simulink model "model1"  (R2023a)
settings: Solver=VariableStepAuto  StartTime=0.0  StopTime=40  RelTol=1e-3
settings Model: Creator=evdokiiagalkina  LastModifiedBy=evdokiiagalkina

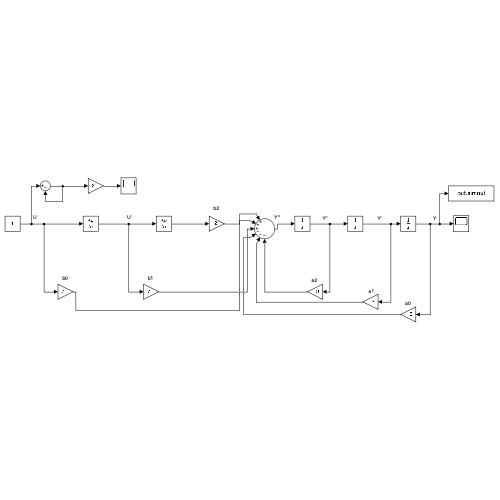
[thumbnail: Simulink's stored preview of the top-level diagram]
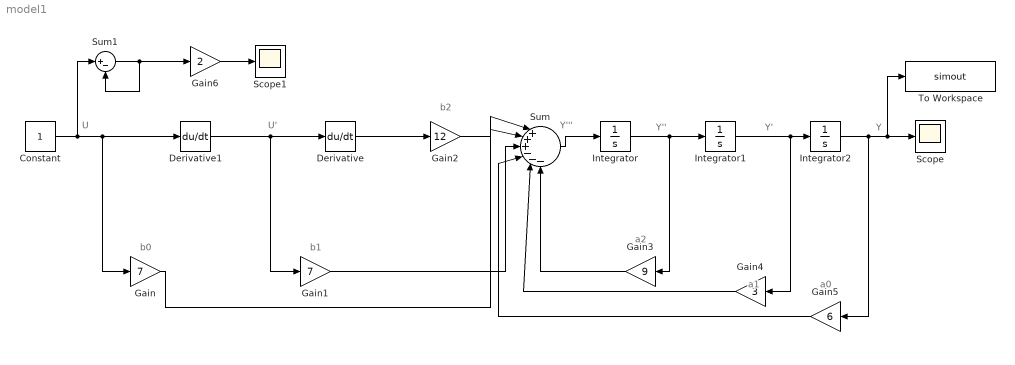
== system model1 ==
  note: Y''
  note: Y'''
  note: U'
  note: b0
  note: U
  note: b1
  note: b2
  note: Y'
  note: Y
  note: a2
  note: a1
  note: a0
  Constant : Constant
  Derivative : Derivative
  Derivative1 : Derivative
  Gain : Gain  Gain=7
  Gain1 : Gain  Gain=7
  Gain2 : Gain  Gain=12
  Gain3 : Gain  Gain=9
  Gain4 : Gain  Gain=3
  Gain5 : Gain  Gain=6
  Gain6 : Gain  Gain=2
  Integrator : Integrator
  Integrator1 : Integrator
  Integrator2 : Integrator
  Scope : Scope
  Scope1 : Scope
  Sum : Sum  Inputs=|+++---
  Sum1 : Sum  Inputs=|+-
  To Workspace : ToWorkspace  VariableName=simout  SaveFormat=Timeseries  SampleTime=-1
  wires:
  Sum/1 -> Integrator/1
  Derivative1/1 -> Derivative/1, Gain1/1
  Derivative/1 -> Gain2/1
  Gain/1 -> Sum/2
  Gain1/1 -> Sum/3
  Gain2/1 -> Sum/1
  Integrator/1 -> Gain3/1, Integrator1/1
  Integrator1/1 -> Gain4/1, Integrator2/1
  Gain3/1 -> Sum/6
  Gain4/1 -> Sum/5
  Gain5/1 -> Sum/4
  Constant/1 -> Sum1/1, Gain/1, Derivative1/1
  Sum1/1 -> Gain6/1, Sum1/2
  Gain6/1 -> Scope1/1
  Integrator2/1 -> Gain5/1, To Workspace/1, Scope/1
